simulink model "AE_315_W2_RL_circuit_charge"  (R2022b)
settings: Solver=VariableStepAuto  StartTime=0.0  StopTime=10.0  RelTol=1e-3
settings Model: Creator=SoftLaptop  LastModifiedBy=SoftLaptop

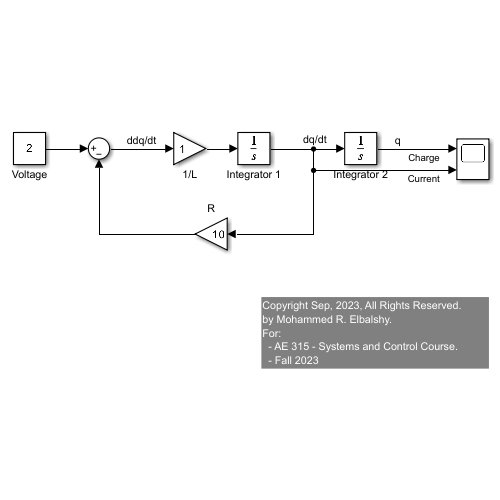
[thumbnail: Simulink's stored preview of the top-level diagram]
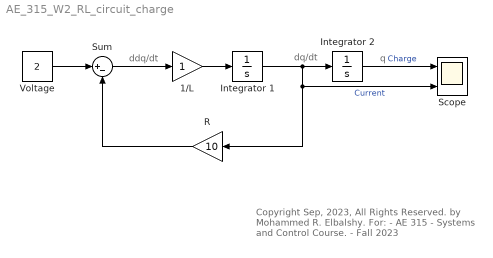
== system AE_315_W2_RL_circuit_charge ==
  note: dq/dt
  note: ddq/dt
  note: q
  note: Copyright Sep, 2023, All Rights Reserved.
      | by Mohammed R. Elbalshy.
      | For:
      | - AE 315 - Systems and Control Course.
      | - Fall 2023
  1/L : Gain
  Integrator 1 : Integrator
  Integrator 2 : Integrator
  R : Gain  Gain=10
  Scope : Scope  NumInputPorts=2
  Sum : Sum  Inputs=|+-
  Voltage : Constant  Value=2
  wires:
  Voltage/1 -> Sum/1
  Sum/1 -> 1/L/1
  1/L/1 -> Integrator 1/1
  Integrator 1/1 -> R/1, Scope/2, Integrator 2/1  "Current"
  R/1 -> Sum/2
  Integrator 2/1 -> Scope/1  "Charge"
